simulink model "Vehicle1"  (R2023b)
settings: Solver=VariableStepAuto  StartTime=0.0  StopTime=1220  RelTol=1e-3
undefined symbols (not defined in the file): DiscIntNeverNeededParam
libraries: qss_tb_library x5
settings Model: Creator=marri  LastModifiedBy=marri

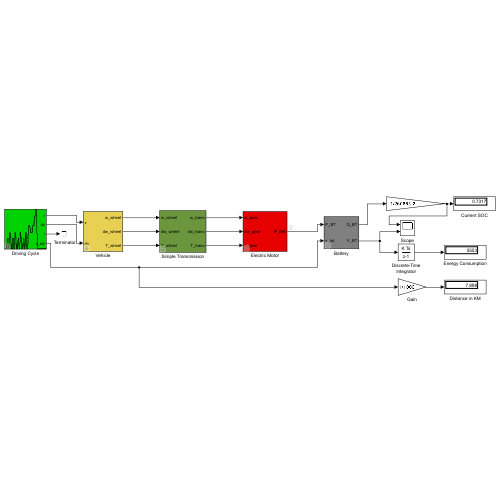
[thumbnail: Simulink's stored preview of the top-level diagram]
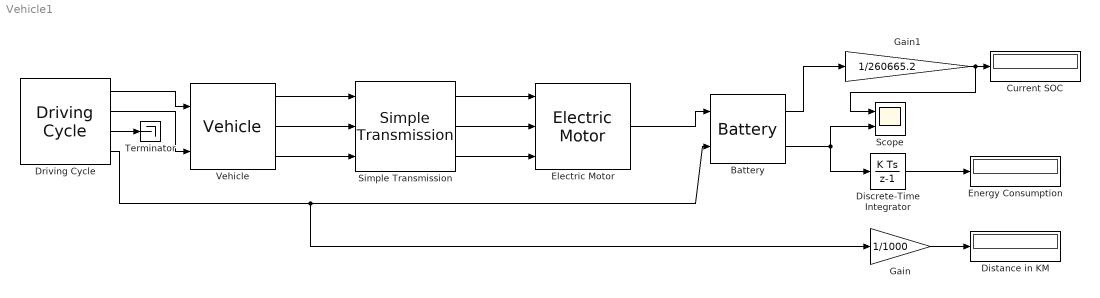
== system Vehicle1 ==
  Battery : qss_tb_library/Energy Buffer/Battery  Tag=battery  I_0=72.407  Q_BT_IC_rel=80  t_ch=20
  Current SOC : Display
  Discrete-Time Integrator : DiscreteIntegrator  SampleTime=-1  ICPrevOutput=DiscIntNeverNeededParam  ICPrevScaledInput=DiscIntNeverNeededParam
  Distance in KM : Display
  Driving Cycle : qss_tb_library/Driving Cycle/Driving Cycle  Tag=cycle  cyclenr=Europe: NEDC  stepsize=1  autostop=on
  Electric Motor : qss_tb_library/Energy Converter/Electric Motor  scale_EM=1  theta_EM=0.1  P_aux=0
  Energy Consumption : Display
  Gain : Gain  Gain=1/1000
  Gain1 : Gain  Gain=1/260665.2
  Scope : Scope  NumInputPorts=2
  Simple Transmission : qss_tb_library/Gear System/Simple Transmission  Tag=simple transmission  gear_ratio=2  e_GT=0.98  P_GT0=50  w_wheel_min=1
  Terminator : Terminator
  Vehicle : qss_tb_library/Vehicle/Vehicle  Tag=vehicle  m_f=191  mt2m_f=5  A_f=0.875  d_wheel=0.233  cw=1.5  mu=0.02
  wires:
  Driving Cycle/1 -> Vehicle/1
  Driving Cycle/3 -> Terminator/1
  Vehicle/1 -> Simple Transmission/1
  Vehicle/2 -> Simple Transmission/2
  Vehicle/3 -> Simple Transmission/3
  Simple Transmission/1 -> Electric Motor/1
  Simple Transmission/3 -> Electric Motor/3
  Simple Transmission/2 -> Electric Motor/2
  Electric Motor/1 -> Battery/1
  Driving Cycle/4 -> Gain/1, Battery/2
  Battery/1 -> Gain1/1
  Battery/2 -> Discrete-Time Integrator/1, Scope/2
  Discrete-Time Integrator/1 -> Energy Consumption/1
  Gain/1 -> Distance in KM/1
  Gain1/1 -> Scope/1, Current SOC/1
  Driving Cycle/2 -> Vehicle/2
